simulink model "InClarkPark"  (R2025b)
settings: Solver=VariableStepAuto  StartTime=0.0  StopTime=10.0  RelTol=1e-3
settings Model: Creator=jff_1  LastModifiedBy=jff_1

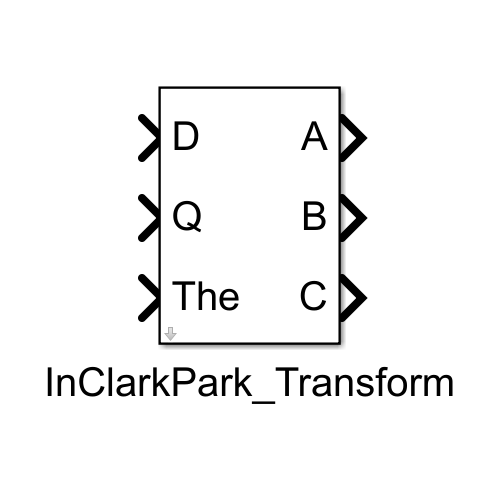
[thumbnail: Simulink's stored preview of the top-level diagram]
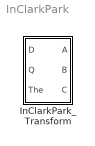
== system InClarkPark ==
  InClarkPark_Transform : Subsystem
      mask help:
      | 本模块实现 dqθ 坐标系到三相自然坐标系 abc 的反 Park 变换。
      |
      | 反 Park 变换用于将同步旋转坐标系下的 d、q 分量，
      | 根据给定的电角度 θ，恢复为三相定子坐标系中的
      | a、b、c 三相量。
      |
      | 该变换常用于矢量控制（FOC）中，
      | 在电流/电压控制器之后，将 dq 控制量转换为三相参考量，
      | 以供逆变器调制与驱动使用。
      mask Help:
      | 本模块实现 dqθ 坐标系到三相自然坐标系 abc 的反 Park 变换。
      | 
      | 反 Park 变换用于将同步旋转坐标系下的 d、q 分量，
      | 根据给定的电角度 θ，恢复为三相定子坐标系中的
      | a、b、c 三相量。
      | 
      | 该变换常用于矢量控制（FOC）中，
      | 在电流/电压控制器之后，将 dq 控制量转换为三相参考量，
      | 以供逆变器调制与驱动使用。
      mask DialogControl ParameterGroupVar Prompt: 参数
      mask Display:
      | % 输入端口
      | port_label('input',1,'D');
      | port_label('input',2,'Q');
      | port_label('input',3,'The');
      | 
      | % 输出端口
      | port_label('output',1,'A');
      | port_label('output',2,'B');
      | port_label('output',3,'C');

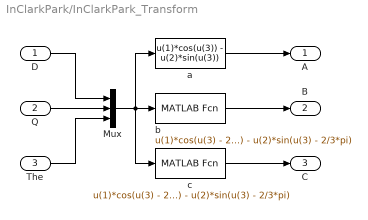
== system InClarkPark/InClarkPark_Transform ==
  D : Inport
  Q : Inport  Port=2
  The : Inport  Port=3
  Mux : Mux  Inputs=3
  a : MATLABFcn  MATLABFcn=u(1)*cos(u(3)) - u(2)*sin(u(3))
  b : MATLABFcn  MATLABFcn=u(1)*cos(u(3) - 2/3*pi) - u(2)*sin(u(3) - 2/3*pi)
  c : MATLABFcn  MATLABFcn=u(1)*cos(u(3) - 2/3*pi) - u(2)*sin(u(3) - 2/3*pi)
  A : Outport
  B : Outport  Port=2
  C : Outport  Port=3
  wires:
  Q/1 -> Mux/2
  Mux/1 -> c/1, a/1, b/1
  The/1 -> Mux/3
  c/1 -> C/1
  a/1 -> A/1
  D/1 -> Mux/1
  b/1 -> B/1
